simulink model "rs_qam"  (R2018b)
settings: Solver=VariableStepAuto  StartTime=0.0  StopTime=53000  RelTol=1e-3
undefined symbols (not defined in the file): K, M, rsgenpoly
libraries: commutil2 x4, commsink2 x2, commblkcod2 x2, commdigbbndam3 x2, commchan3 x1, dspmathops x1, commrandsrc3 x1
settings Model: Creator=Tejasvi  LastModifiedBy=Tejasvi

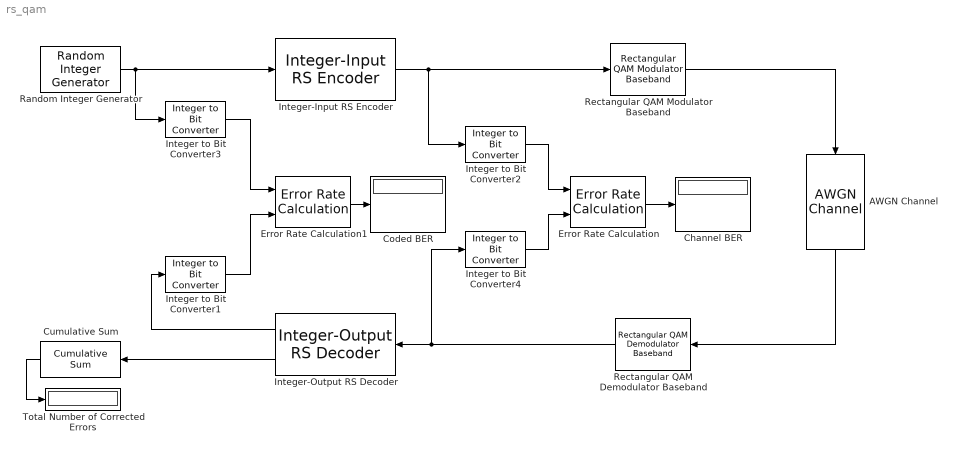
== system rs_qam ==
  AWGN Channel : commchan3/AWGN Channel  InputProcessing=Columns as channels (frame based)  seed=67  noiseMode="Signal to noise ratio  (Eb/No)"  EbNodB=10*log10(K/(M-1)) + 15  EsNodB=10  SNRdB=10  bitsPerSym=B  Ps=45  Tsym=1  variance=1
  Channel BER : Display
  Coded BER : Display
  Cumulative Sum : dspmathops/Cumulative Sum  dim=Channels (running sum)  InputProcessing=Columns as channels (frame based)  reset_popup=None  roundingMode=Floor  overflowMode=off  outputDataTypeStr=Inherit: Same as accumulator  outputMin=[]  outputMax=[]  outputLastDataTypeStr=Inherit: Same as accumulator
      settings: SourceProductName=DSP System Toolbox
  Error Rate Calculation : commsink2/Error Rate Calculation  N=0  st_delay=0  cp_mode=Entire frame  subframe=[]  PMode=Port  WsName=ErrorVec  RsMode2=off  stop=off  numErr=100  maxBits=1e6
  Error Rate Calculation1 : commsink2/Error Rate Calculation  N=0  st_delay=0  cp_mode=Entire frame  subframe=[]  PMode=Port  WsName=ErrorVec  RsMode2=off  stop=off  numErr=100  maxBits=1e6
  Integer to Bit Converter{1..4} (4 alike) : commutil2/Integer to Bit Converter  nbits=B  signedInputValues=Unsigned  bitOrder=MSB first  outDtype=Inherit via internal rule
  Integer-Input RS Encoder : commblkcod2/Integer-Input RS Encoder  n=M-1  k=K  specShortening=off  shortenedK=3  specGenPoly=off  genPoly=rsgenpoly(7, 3, [], [], 'double')  specPrimPoly=off  prPoly='X^3 + X + 1'  specPuncture=off  punctVec=[ones(2,1); zeros(2,1)]
      settings: SourceProductName=Communications System Toolbox  SourceProductBaseCode=CM
  Integer-Output RS Decoder : commblkcod2/Integer-Output RS Decoder  n=M-1  k=K  specShortening=off  shortenedK=3  specGenPoly=off  genPoly=rsgenpoly(7, 3, [], [], 'double')  specPrimPoly=off  prPoly='X^3 + X + 1'  specPuncture=off  punctVec=[ones(2,1); zeros(2,1)]  specErasurePort=off  showNumErr=on
      settings: SourceProductName=Communications System Toolbox  SourceProductBaseCode=CM
  Random Integer Generator : commrandsrc3/Random Integer Generator  SetSize=M  SeedSource=Auto  Seed=0  SampleTime=1  SamplesPerFrame=K  OutputDataType=double  SimulateUsing=Interpreted execution
  Rectangular QAM Demodulator Baseband : commdigbbndam3/Rectangular QAM Demodulator Baseband  M=M  OutType=Integer  DecType=Hard decision  VarSource=Dialog  Variance=1  Dec=Gray  Mapping=[0:15]  PowType=Min. distance between symbols  MinDist=2  AvgPow=1  PeakPow=1  Ph=0  outDtype1=Inherit via internal rule  outDtype2=Inherit via internal rule  derotateFactorWordLen=16  derotateFactorDataTypeStr=Inherit: Same word length as input  derotateFactorLastDataTypeStr=Inherit: Same word length as input  denormFactorWordLen=16  denormFactorDataTypeStr=Inherit: Same word length as input  denormFactorLastDataTypeStr=Inherit: Same word length as input  prodOutWordLen=32  prodOutOverflowMode=Wrap  prodOutRoundingMode=Floor  prodOutOvFlMode=off  prodOutOvFlModeLastStrValue=off  sumWordLen=32
  Rectangular QAM Modulator Baseband : commdigbbndam3/Rectangular QAM Modulator Baseband  M=M  InType=Integer  Enc=Gray  Mapping=[0:15]  PowType=Min. distance between symbols  MinDist=2  AvgPow=1  PeakPow=1  Ph=0  outDtype=double  outWordLen=16  outUDDataType=sfix(16)  outFracLenMode=Best precision  outFracLen=15  outDataTypeStr=double  outLastDataTypeStr=double
  "Total Number of Corrected Errors " : Display
  wires:
  Error Rate Calculation/1 -> Channel BER/1
  AWGN Channel/1 -> Rectangular QAM Demodulator Baseband/1
  Cumulative Sum/1 -> "Total Number of Corrected Errors "/1
  Integer-Output RS Decoder/2 -> Cumulative Sum/1
  Rectangular QAM Demodulator Baseband/1 -> Integer to Bit Converter4/1, Integer-Output RS Decoder/1
  Integer-Input RS Encoder/1 -> Integer to Bit Converter2/1, Rectangular QAM Modulator Baseband/1
  Error Rate Calculation1/1 -> Coded BER/1
  Integer to Bit Converter3/1 -> Error Rate Calculation1/1
  Integer to Bit Converter1/1 -> Error Rate Calculation1/2
  Integer to Bit Converter4/1 -> Error Rate Calculation/2
  Integer to Bit Converter2/1 -> Error Rate Calculation/1
  Random Integer Generator/1 -> Integer to Bit Converter3/1, Integer-Input RS Encoder/1
  Integer-Output RS Decoder/1 -> Integer to Bit Converter1/1
  Rectangular QAM Modulator Baseband/1 -> AWGN Channel/1
